simulink library "aruco_nano_detector_Lib"  (R2022a)
settings: Solver=FixedStepAuto  StartTime=0.0  StopTime=10.0  RelTol=1e-3
PostLoadFcn:
  | set_param(gcs, 'CustomCodeGlobalsAsFunctionIO', 'on');
undefined symbols (not defined in the file): Image, Mat
libraries: opencvConverterBlockset x8
settings Model: Creator=Rafael  LastModifiedBy=Rafael
settings OptimizationCC: ZeroExternalMemoryAtStartup=off  ZeroInternalMemoryAtStartup=off
settings SFSimCC: SimUserLibraries=$SLCC.Utils.GetMLBuiltinOpenCVLibs$  DefaultCustomCodeFunctionArrayLayout=Row-major  CustomCodeUndefinedFunction=UseInterfaceOnly  CustomCodeGlobalsAsFunctionIO=on  SimTargetLang=C++
settings SFSimCC: SimCustomHeaderCode=|
  | #include  "aruco_nano_detector_Wrapper_sim.hpp"
  | #include  "CVDeepCopyHelper.hpp"
settings SFSimCC: SimUserSources=|
  | .\aruco_nano_detector.cpp
  | aruco_nano_detector_Wrapper_sim.cpp
  | CVDeepCopyHelper.cpp
settings SFSimCC: SimUserIncludeDirs=|
  | "$matlabroot$/toolbox/vision/builtins/src/ocvcg/opencv/include"
  | $matlabshared.supportpkg.getSupportPackageRoot()$/toolbox/simulink/supportpackages/simulinkopencv/converterBlockSet
settings RTWCC: CustomHeaderCode="#include  \"aruco_nano_detector_Wrapper_cg.hpp\""  CustomInclude="\"$matlabroot$/toolbox/vision/builtins/src/ocvcg/opencv/include\""  CustomLibrary=$SLCC.Utils.GetMLBuiltinOpenCVLibs$  TargetLang=C++
settings RTWCC: CustomSource=|
  | .\aruco_nano_detector.cpp
  | aruco_nano_detector_Wrapper_cg.cpp
settings GRTTargetCC: TargetLangStandard=C++11 (ISO)  CodeInterfacePackaging=C++ class

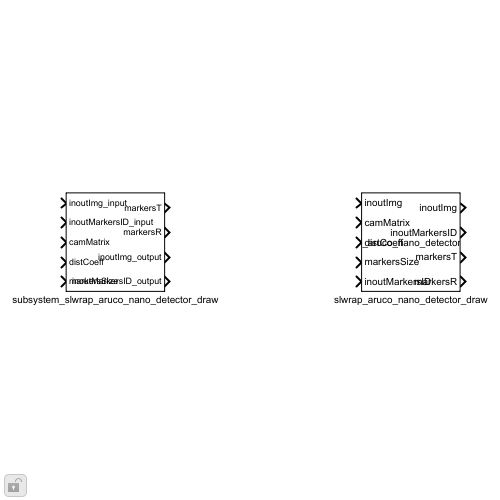
[thumbnail: Simulink's stored preview of the top-level diagram]
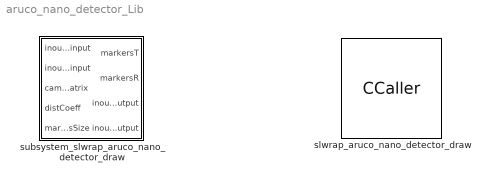
== system aruco_nano_detector_Lib ==
  slwrap_aruco_nano_detector_draw : CCaller  FunctionName=slwrap_aruco_nano_detector_draw  PortSpecificationStruct="%)30     .    P P   8    (     @         %    \"     <    !     0         %  0 \"0    $    _    07)G3F%M90  4&]R=$YA;64 4V-O<&4     26YD97@     5'EP90      4VEZ90      27-';&]B86P   X    X    !@    @    $          4    (     0    @    !         !     (    :6YO=71);6<.    .     8    (    !          %    \"     $    (     0         0    \"    &EN;W5T26UG#@   $     &    \"     0         !0    @    !  ...(+4027 chars)"
  subsystem_slwrap_aruco_nano_detector_draw : Subsystem  mask{mRows1=4, mRows2=4, matRows3=1080, matCols3=1920, matChannels3=3, mUnderlyingType3=uint8, mIsImage3=on, mRows4=4}
      mask prompts: mRows1 "Rows"; mRows2 "Rows"; matRows3 "Rows"; matCols3 "Columns"; matChannels3 "Channels"; mUnderlyingType3 "Underlying Type"; mIsImage3 "is Image"; mRows4 "Rows"
      mask Callback mRows1: conv = [gcb  '/FromOpenCV']; rows = get_param(gcb,'mRows1');  set_param(conv, 'rows', rows);
      mask Callback mRows2: conv = [gcb  '/FromOpenCV1']; rows = get_param(gcb,'mRows2');  set_param(conv, 'rows', rows);
      mask Callback matRows3: conv = [gcb  '/FromOpenCV2']; rows = get_param(gcb,'matRows3'); set_param(conv, 'rows', rows);
      mask Callback matCols3: conv = [gcb  '/FromOpenCV2']; cols = get_param(gcb,'matCols3'); set_param(conv, 'columns', cols);
      mask TypeOptions matChannels3: 1 | 2 | 3 | 4
      mask Callback matChannels3: conv = [gcb  '/FromOpenCV2']; channels = get_param(gcb,'matChannels3'); set_param(conv, 'channels', channels);
      mask TypeOptions mUnderlyingType3: uint8 | int8 | uint16 | int16 | int32 | single | double
      mask Callback mUnderlyingType3: conv = [gcb  '/FromOpenCV2']; underlyingdatatype = get_param(gcb,'mUnderlyingType3'); set_param(conv, 'underlyingDataType', underlyingdatatype);
      mask Callback mIsImage3:
      | conv = gcb + "/" + "FromOpenCV2"; isimage = get_param(gcb,"mIsImage3");
      | if isimage == "off"
      | set_param(conv, "dataType", "Mat");
      | mMask = Simulink.Mask.get(gcb);
      | mMask.Parameters(3).TypeOptions = {"1";"2";"3";"4"};
      | else
      | set_param(conv, "dataType", "Mat-Image");
      | mMask = Simulink.Mask.get(gcb);
      | mMask.Parameters(3).TypeOptions = {"1";"3"};
      | end
      mask Callback mRows4: conv = [gcb  '/FromOpenCV3']; rows = get_param(gcb,'mRows4');  set_param(conv, 'rows', rows);
      mask DialogControl tab1 Prompt: std::vector<cv::Point3d> markersT
      mask DialogControl tab2 Prompt: std::vector<cv::Point3d> markersR
      mask DialogControl tab3 Prompt: cv::Mat inoutImg
      mask DialogControl tab4 Prompt: std::vector<cv::Point2i> inoutMarkersID

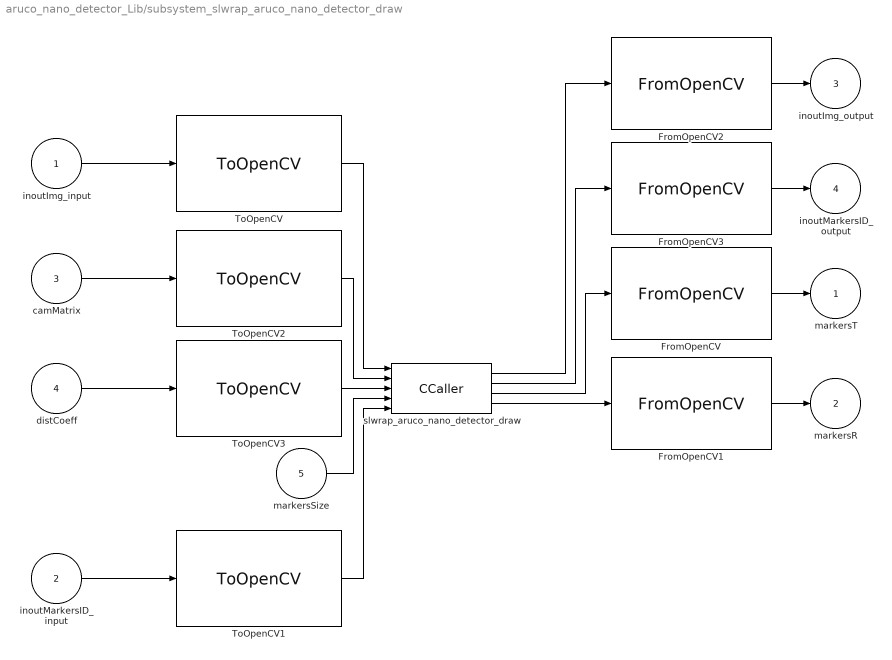
== system aruco_nano_detector_Lib/subsystem_slwrap_aruco_nano_detector_draw ==
  inoutImg_input : Inport
  inoutMarkersID_input : Inport  Port=2
  camMatrix : Inport  Port=3
  distCoeff : Inport  Port=4
  markersSize : Inport  Port=5
  FromOpenCV : opencvConverterBlockset/FromOpenCV  dataType=vector<Point3d>  rows=1  columns=1  channels=1  underlyingDataType=uint8  arrayLayout=Column-major  colorFormat=RGB
      settings: SourceProductBaseCode=SM_OPENCV
  FromOpenCV1 : opencvConverterBlockset/FromOpenCV  dataType=vector<Point3d>  rows=1  columns=1  channels=1  underlyingDataType=uint8  arrayLayout=Column-major  colorFormat=RGB
      settings: SourceProductBaseCode=SM_OPENCV
  FromOpenCV2 : opencvConverterBlockset/FromOpenCV  dataType=Mat-Image  rows=1080  columns=1920  channels=3  underlyingDataType=uint8  arrayLayout=Column-major  colorFormat=RGB
      settings: SourceProductBaseCode=SM_OPENCV
  FromOpenCV3 : opencvConverterBlockset/FromOpenCV  dataType=vector<Point2i>  rows=1  columns=1  channels=1  underlyingDataType=uint8  arrayLayout=Column-major  colorFormat=RGB
      settings: SourceProductBaseCode=SM_OPENCV
  ToOpenCV : opencvConverterBlockset/ToOpenCV  dataType=Mat-Image
      settings: SourceProductBaseCode=SM_OPENCV
  ToOpenCV1 : opencvConverterBlockset/ToOpenCV  dataType=vector<Point2i>
      settings: SourceProductBaseCode=SM_OPENCV
  ToOpenCV2 : opencvConverterBlockset/ToOpenCV  dataType=Mat-Image
      settings: SourceProductBaseCode=SM_OPENCV
  ToOpenCV3 : opencvConverterBlockset/ToOpenCV  dataType=Mat-Image
      settings: SourceProductBaseCode=SM_OPENCV
  slwrap_aruco_nano_detector_draw : CCaller  FunctionName=slwrap_aruco_nano_detector_draw  PortSpecificationStruct="%)30     .    P P   8    (     @         %    \"     <    !     0         %  0 \"0    $    _    07)G3F%M90  4&]R=$YA;64 4V-O<&4     26YD97@     5'EP90      4VEZ90      27-';&]B86P   X    X    !@    @    $          4    (     0    @    !         !     (    :6YO=71);6<.    .     8    (    !          %    \"     $    (     0         0    \"    &EN;W5T26UG#@   $     &    \"     0         !0    @    !  ...(+4027 chars)"
  markersT : Outport
  markersR : Outport  Port=2
  inoutImg_output : Outport  Port=3
  inoutMarkersID_output : Outport  Port=4
  wires:
  ToOpenCV1/1 -> slwrap_aruco_nano_detector_draw/5
  ToOpenCV3/1 -> slwrap_aruco_nano_detector_draw/3
  markersSize/1 -> slwrap_aruco_nano_detector_draw/4
  FromOpenCV1/1 -> markersR/1
  distCoeff/1 -> ToOpenCV3/1
  ToOpenCV2/1 -> slwrap_aruco_nano_detector_draw/2
  camMatrix/1 -> ToOpenCV2/1
  inoutMarkersID_input/1 -> ToOpenCV1/1
  FromOpenCV3/1 -> inoutMarkersID_output/1
  slwrap_aruco_nano_detector_draw/3 -> FromOpenCV/1
  slwrap_aruco_nano_detector_draw/2 -> FromOpenCV3/1
  inoutImg_input/1 -> ToOpenCV/1
  ToOpenCV/1 -> slwrap_aruco_nano_detector_draw/1
  FromOpenCV2/1 -> inoutImg_output/1
  slwrap_aruco_nano_detector_draw/1 -> FromOpenCV2/1
  slwrap_aruco_nano_detector_draw/4 -> FromOpenCV1/1
  FromOpenCV/1 -> markersT/1
